simulink model "kinematic_control"  (R2015b)
settings: Solver=FixedStepAuto  StartTime=0.0  StopTime=20  FixedStep=0.01  MaxStep=0.01  RelTol=1e-3
values from neighbouring files (symbols this model uses):
  Kd = 0    [KINEMATIC_VEHICLE_CONTROL.m]
  Ki = 0    [KINEMATIC_VEHICLE_CONTROL.m]
  Kp = 4    [KINEMATIC_VEHICLE_CONTROL.m]
  Lf = 1    [KINEMATIC_MOTION_PLANNER.m]    (also in KINEMATIC_MOTION_PLANNER2.m; KINEMATIC_STEP_MPC.m; KINEMATIC_VEHICLE_CONTROL.m; KINEMATIC_VEHICLE_SIM.m)
  Lr = 1    [KINEMATIC_MOTION_PLANNER.m]    (also in KINEMATIC_MOTION_PLANNER2.m; KINEMATIC_STEP_MPC.m; KINEMATIC_VEHICLE_CONTROL.m; KINEMATIC_VEHICLE_SIM.m)
  Psi0 = 0    [KINEMATIC_MOTION_PLANNER.m]    (also in KINEMATIC_MOTION_PLANNER2.m; KINEMATIC_STEP_MPC.m; KINEMATIC_VEHICLE_CONTROL.m; KINEMATIC_VEHICLE_SIM.m)
  R = [ct -st;st ct]    [DrawRectangle.m]    (also in KINEMATIC_VEHICLE_CONTROL.m = 8)
  V = 1    [KINEMATIC_MOTION_PLANNER.m]    (also in KINEMATIC_MOTION_PLANNER2.m; KINEMATIC_STEP_MPC.m; KINEMATIC_VEHICLE_CONTROL.m; KINEMATIC_VEHICLE_SIM.m = 5)
  X0 = 0    [KINEMATIC_MOTION_PLANNER.m]    (also in KINEMATIC_MOTION_PLANNER2.m; KINEMATIC_STEP_MPC.m; KINEMATIC_VEHICLE_CONTROL.m; KINEMATIC_VEHICLE_SIM.m)
  Y0 = 0    [KINEMATIC_MOTION_PLANNER.m]    (also in KINEMATIC_MOTION_PLANNER2.m; KINEMATIC_STEP_MPC.m; KINEMATIC_VEHICLE_CONTROL.m; KINEMATIC_VEHICLE_SIM.m)
settings Model: Creator=gebruiker  LastModifiedBy=gebruiker

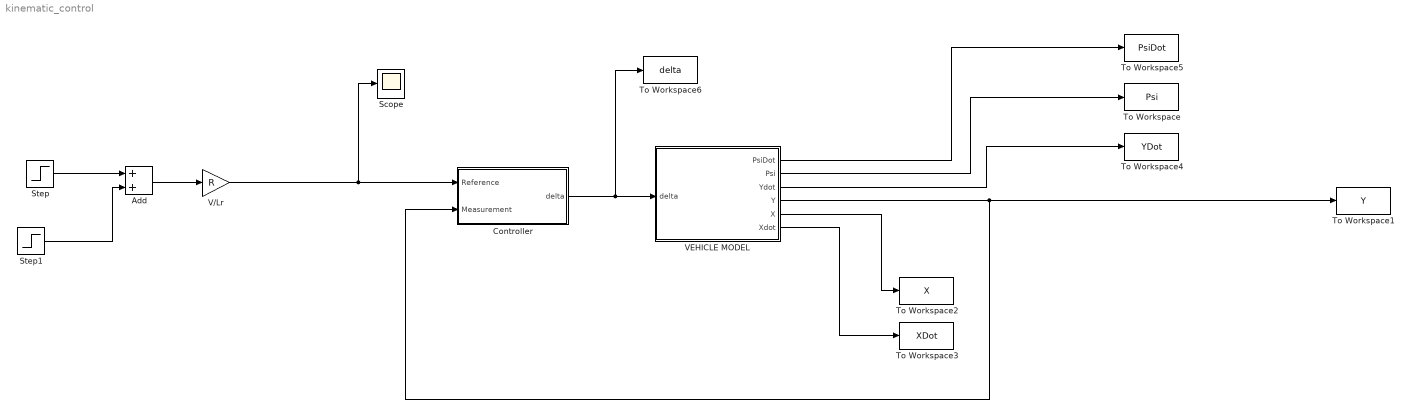
== system kinematic_control ==
  Add : Sum
  Controller : Subsystem
  Scope : Scope
  Step : Step  SampleTime=0
  Step1 : Step  Time=5  After=0  SampleTime=0
  To Workspace : ToWorkspace  VariableName=Psi  SaveFormat=Structure With Time  SampleTime=-1
  To Workspace1 : ToWorkspace  VariableName=Y  SaveFormat=Structure With Time  SampleTime=-1
  To Workspace2 : ToWorkspace  VariableName=X  SaveFormat=Structure With Time  SampleTime=-1
  To Workspace3 : ToWorkspace  VariableName=XDot  SaveFormat=Structure With Time  SampleTime=-1
  To Workspace4 : ToWorkspace  VariableName=YDot  SaveFormat=Structure With Time  SampleTime=-1
  To Workspace5 : ToWorkspace  VariableName=PsiDot  SaveFormat=Structure With Time  SampleTime=-1
  To Workspace6 : ToWorkspace  VariableName=delta  SaveFormat=Structure With Time  SampleTime=-1
  V/Lr : Gain  Gain=R
  VEHICLE MODEL : Subsystem
  wires:
  VEHICLE MODEL/1(PsiDot) -> To Workspace5/1
  VEHICLE MODEL/2(Psi) -> To Workspace/1
  VEHICLE MODEL/3(Ydot) -> To Workspace4/1
  VEHICLE MODEL/4(Y) -> To Workspace1/1, Controller/2(Measurement)
  VEHICLE MODEL/5(X) -> To Workspace2/1
  VEHICLE MODEL/6(Xdot) -> To Workspace3/1
  Controller/1(delta) -> To Workspace6/1, VEHICLE MODEL/1("delta ")
  V/Lr/1 -> Scope/1, Controller/1(Reference)
  Step/1 -> Add/1
  Step1/1 -> Add/2
  Add/1 -> V/Lr/1

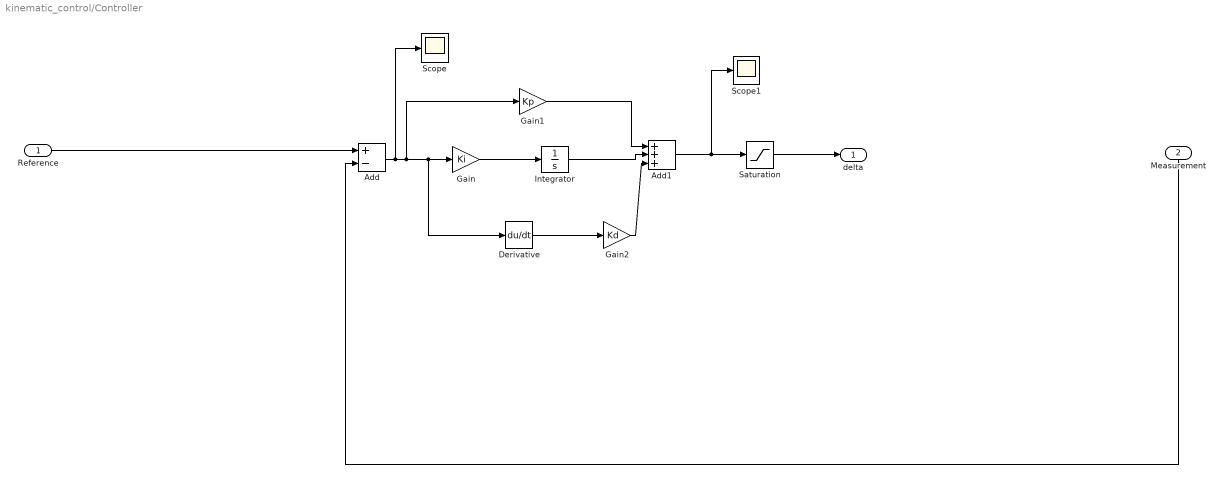
== system kinematic_control/Controller ==
  Reference : Inport
  Measurement : Inport  Port=2
  Add : Sum  Inputs=+-
  Add1 : Sum  Inputs=+++
  Derivative : Derivative
  Gain : Gain  Gain=Ki
  Gain1 : Gain  Gain=Kp
  Gain2 : Gain  Gain=Kd
  Integrator : Integrator  LimitOutput=on  UpperSaturationLimit=pi/6  LowerSaturationLimit=-pi/6
  Saturation : Saturate  UpperLimit=pi/6  LowerLimit=-pi/6
  Scope : Scope
  Scope1 : Scope
  delta : Outport
  wires:
  Add/1 -> Scope/1, Gain1/1, Derivative/1, Gain/1
  Measurement/1 -> Add/2
  Reference/1 -> Add/1
  Gain/1 -> Integrator/1
  Gain1/1 -> Add1/1
  Integrator/1 -> Add1/2
  Add1/1 -> Scope1/1, Saturation/1
  Saturation/1 -> delta/1
  Derivative/1 -> Gain2/1
  Gain2/1 -> Add1/3

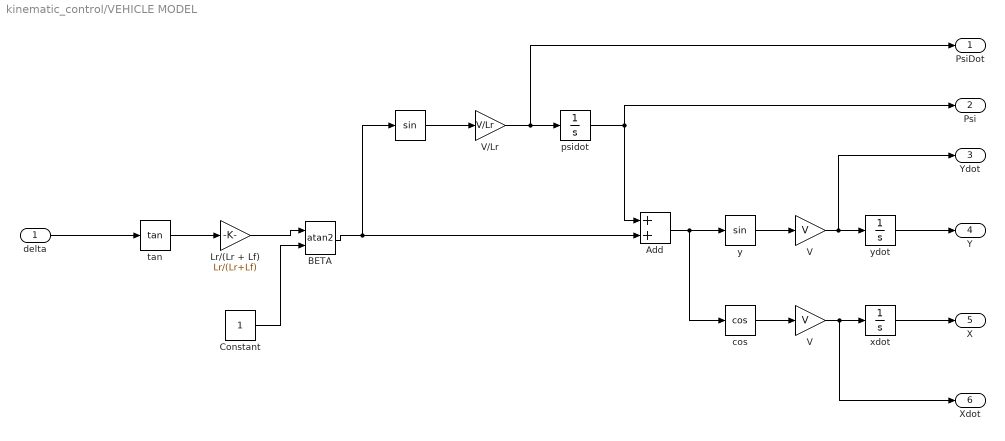
== system kinematic_control/VEHICLE MODEL ==
  "delta " : Inport
  " " : Trigonometry
  Add : Sum
  BETA : Trigonometry  Operator=atan2
  Constant : Constant
  Lr/(Lr + Lf) : Gain  Gain=Lr/(Lr+Lf)
  V : Gain  Gain=V
  "V " : Gain  Gain=V
  V/Lr : Gain  Gain=V/Lr
  cos : Trigonometry  Operator=cos
  psidot : Integrator  InitialCondition=Psi0
  "tan " : Trigonometry  Operator=tan
  xdot : Integrator  InitialCondition=X0
  y : Trigonometry
  ydot : Integrator  InitialCondition=Y0
  PsiDot : Outport
  Psi : Outport  Port=2
  Ydot : Outport  Port=3
  Y : Outport  Port=4
  X : Outport  Port=5
  Xdot : Outport  Port=6
  wires:
  V/1 -> Ydot/1, ydot/1
  Lr/(Lr + Lf)/1 -> BETA/1
  BETA/1 -> Add/2, " "/1
  "V "/1 -> Xdot/1, xdot/1
  Add/1 -> cos/1, y/1
  xdot/1 -> X/1
  ydot/1 -> Y/1
  psidot/1 -> Psi/1, Add/1
  "delta "/1 -> "tan "/1
  V/Lr/1 -> PsiDot/1, psidot/1
  y/1 -> V/1
  " "/1 -> V/Lr/1
  "tan "/1 -> Lr/(Lr + Lf)/1
  cos/1 -> "V "/1
  Constant/1 -> BETA/2
